simulink model "mcb_pmsm_foc_sensorless_dyno_f28379d"  (R2024b)
settings: Solver=FixedStepDiscrete  StartTime=0.0  StopTime=6  RelTol=1e-3  EnableMultiTasking=on
InitFcn:
  | mcb_pmsm_foc_sensorless_dyno_f28379d_datascript;
model workspace (MAT data in the model file):
  encoderResolution = 2000
  hallOffset = '0.5'
  indexOffset = 850
  polePairs = '4'
undefined symbols (not defined in the file or in its folder): acceleration, dataType, Down, GPTRIP1SEL, GPTRIP2SEL, inverter_motor1, inverter_motor2, PI_params_motor1, PI_params_motor2, pmsm_motor1, pmsm_motor2, PU_System_motor1, PU_System_motor2, PWM_frequency, SlidFCS_params, Speed_openLoop_PU, T_Ref_openLoop, target, Ts, Ts_motor, Ts_simulink, Ts_speed, TZ1, TZ2, Up, Vd_Ref_openLoop_PU
libraries: mcbcontrolslib x20, c2802xlib x14, simulink x8, c280xlib x7, slpidlib x5, c2837xDlib x5, mcbpositiondecoderlib x4, svdschedulerlib x3, mcbsensorlessestimatorlib x2, mcbpmsmnonlinearlib x2, autolibpmsmexterior x2, mcbplantlib x2
(part 1 of 4)
settings Model: ExtModeTrigDuration=8  Creator=The MathWorks, Inc.  LastModifiedBy=Eleonora
settings SolverCC: AlgebraicLoopSolver=TrustRegion
settings DataIOCC: LimitDataPoints=on  SaveFormat=Array  SaveOutput=off  SaveTime=off  ReturnWorkspaceOutputs=off
settings OptimizationCC: DefaultParameterBehavior=Inlined  DefaultUnderspecifiedDataType=single  OptimizeBlockIOStorage=off  BufferReuse=off  GlobalBufferReuse=off  ExpressionFolding=off  ExpressionDepthLimit=2147483647  LocalBlockOutputs=off  InitFltsAndDblsToZero=on  NoFixptDivByZeroProtection=on  EfficientFloat2IntCast=on  EfficientMapNaN2IntZero=off  LifeSpan=Inf  MaxStackSize=1024  OptimizeDataStoreBuffers=off  BusAssignmentInplaceUpdate=off  DenormalBehavior=FlushToZero  EfficientTunableParamExpr=on
settings DebuggingCC: ReadBeforeWriteMsg=DisableAll  WriteAfterWriteMsg=DisableAll  WriteAfterReadMsg=DisableAll  CheckSSInitialOutputMsg=off  SolverPrmCheckMsg=warning  InheritedTsInSrcMsg=none  MultiTaskDSMMsg=none  MultiTaskCondExecSysMsg=none  TasksWithSamePriorityMsg=none  SigSpecEnsureSampleTimeMsg=none  IntegerOverflowMsg=none  ParameterPrecisionLossMsg=none  FcnCallInpInsideContextMsg=warning  UnconnectedInputMsg=warning  UnconnectedOutputMsg=warning  UnconnectedLineMsg=warning  AllowSymbolicDim=off  StateNameClashWarn=warning  SFUnexpectedBacktrackingDiag=warning  SFNoUnconditionalDefaultTransitionDiag=warning  SFExecutionAtInitializationDiag=none  IntegerSaturationMsg=none  ArithmeticOperatorsInVariantConditions=warning
settings HardwareCC: ProdBitPerChar=16  ProdBitPerInt=16  ProdBitPerPointer=32  ProdBitPerSizeT=32  ProdBitPerPtrDiffT=32  ProdLargestAtomicInteger=Integer  ProdLargestAtomicFloat=None  ProdWordSize=16  ProdLongLongMode=on  ProdHWDeviceType=Texas Instruments->C2000  TargetBitPerChar=16  TargetBitPerInt=16  TargetBitPerPointer=16  TargetLargestAtomicInteger=Integer  TargetIntDivRoundTo=Zero  TargetEndianess=LittleEndian  TargetWordSize=16  TargetHWDeviceType=TI C2000
settings ModelReferenceCC: EnableRefExpFcnMdlSchedulingChecks=on  PropagateSignalLabelsOutOfModel=off
settings SFSimCC: SimUseLocalCustomCode=off  MATLABDynamicMemAlloc=off  CustomCodeUndefinedFunction=UseInterfaceOnly
settings RTWCC: Description=Embedded Coder  SystemTargetFile=ert.tlc  HardwareBoard=TI Delfino F28379D LaunchPad  TemplateMakefile=ert_default_tmf  GenerateReport=on  RTWUseLocalCustomCode=off  CustomHeaderCode="#include \"F2837xD_Ipc_drivers.h\""  Toolchain=Texas Instruments Code Composer Studio (C2000)  IncludeHyperlinkInReport=on  LaunchReport=on  GenerateTraceInfo=on  GenerateTraceReport=on  GenerateTraceReportSl=on  GenerateTraceReportSf=on  GenerateTraceReportEml=on  GPUComputeCapability=3.5  DLArmComputeVersion=19.05
settings CodeAppCC: IgnoreCustomStorageClasses=off  CustomSymbolStrType=$N$R$M  StateflowObjectComments=on  InternalIdentifier=Classic
settings ERTTargetCC: CodeReplacementLibrary=TI C28x  MultiwordLength=2048  ExtModeStaticAllocSize=10000  InlinedParameterPlacement=Hierarchical  ConvertIfToSwitch=off  SuppressUnreachableDefaultCases=off  MemSecPackage=tic2000demospkg  DynamicArrayContainerType=coder::array
settings ConfigComp: CovMetricSettings=dw  CovSaveCumulativeToWorkspaceVar=on  CovSaveSingleToWorkspaceVar=on  CovExternalEMLEnable=off  CovSFcnEnable=off

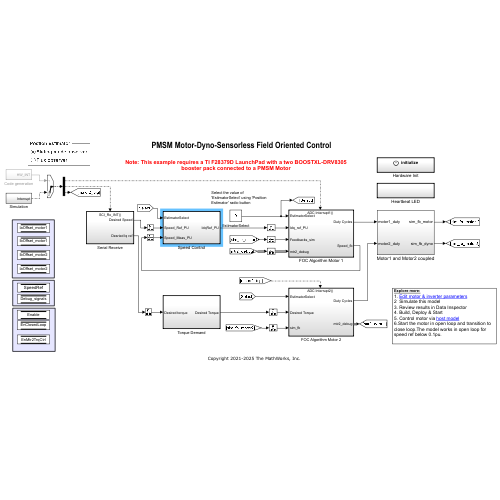
[thumbnail: Simulink's stored preview of the top-level diagram]
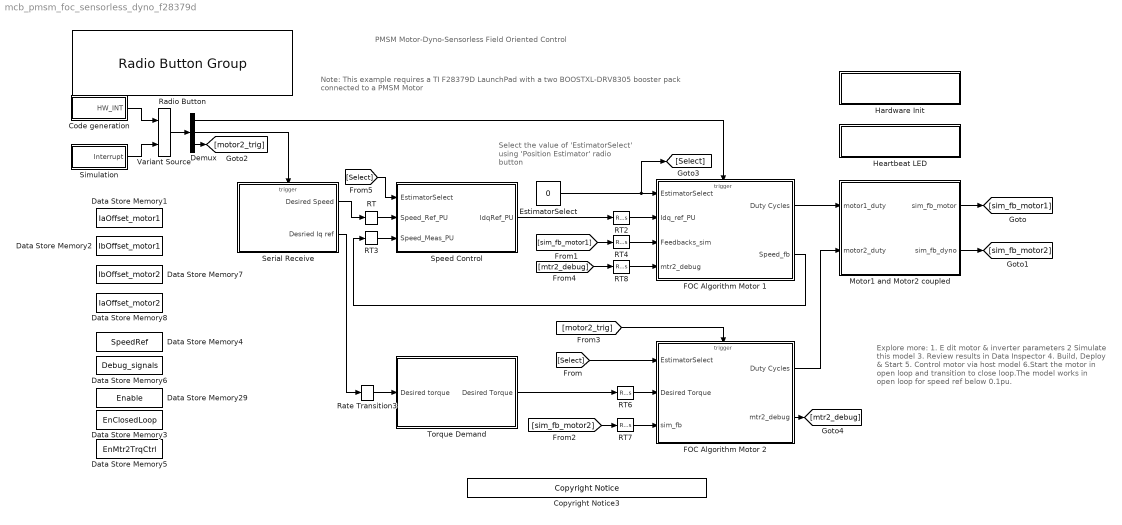
== system mcb_pmsm_foc_sensorless_dyno_f28379d ==
  note: PMSM Motor-Dyno-Sensorless Field Oriented Control
  note: Note: This example requires a TI F28379D LaunchPad with a two BOOSTXL-DRV8305
      | booster pack connected to a PMSM Motor
  note: Explore more:
      | 1. E dit motor & inverter parameters
      | 2 Simulate this model
      | 3. Review results in Data Inspector
      | 4. Build, Deploy & Start
      | 5. Control motor via host model
      | 6.Start the motor in open loop and transition to close loop.The model works in open loop for speed ref below 0.1pu.
  note: Select the value of 'EstimatorSelect' using 'Position Estimator' radio button
  Code generation : Subsystem
  Copyright Notice3 : demo_controls/Copyright Notice  year=2021  prod=tic2000
  Data Store Memory1 : DataStoreMemory  DataStoreName=IaOffset_motor1  ReadBeforeWriteMsg=warning  WriteAfterWriteMsg=warning  WriteAfterReadMsg=warning  InitialValue=inverter_motor1.CtSensAOffset  ShowAdditionalParam=off  OutDataTypeStr=uint16
  Data Store Memory2 : DataStoreMemory  DataStoreName=IbOffset_motor1  ReadBeforeWriteMsg=warning  WriteAfterWriteMsg=warning  WriteAfterReadMsg=warning  InitialValue=inverter_motor1.CtSensBOffset  ShowAdditionalParam=off  OutDataTypeStr=uint16
  Data Store Memory29 : DataStoreMemory  DataStoreName=Enable  ReadBeforeWriteMsg=warning  WriteAfterWriteMsg=warning  WriteAfterReadMsg=warning  ShowAdditionalParam=off  OutDataTypeStr=boolean
  Data Store Memory3 : DataStoreMemory  DataStoreName=EnClosedLoop  ReadBeforeWriteMsg=warning  WriteAfterWriteMsg=warning  WriteAfterReadMsg=warning  ShowAdditionalParam=off  OutDataTypeStr=boolean
  Data Store Memory4 : DataStoreMemory  DataStoreName=SpeedRef  InitialValue=0.1  ShowAdditionalParam=off
  Data Store Memory5 : DataStoreMemory  DataStoreName=EnMtr2TrqCtrl  ReadBeforeWriteMsg=warning  WriteAfterWriteMsg=warning  WriteAfterReadMsg=warning  ShowAdditionalParam=off  OutDataTypeStr=boolean
  Data Store Memory6 : DataStoreMemory  DataStoreName=Debug_signals  ReadBeforeWriteMsg=warning  WriteAfterWriteMsg=warning  WriteAfterReadMsg=warning  InitialValue=5  ShowAdditionalParam=off  OutDataTypeStr=uint16
  Data Store Memory7 : DataStoreMemory  DataStoreName=IbOffset_motor2  ReadBeforeWriteMsg=warning  WriteAfterWriteMsg=warning  WriteAfterReadMsg=warning  InitialValue=inverter_motor2.CtSensBOffset  ShowAdditionalParam=off  OutDataTypeStr=uint16
  Data Store Memory8 : DataStoreMemory  DataStoreName=IaOffset_motor2  ReadBeforeWriteMsg=warning  WriteAfterWriteMsg=warning  WriteAfterReadMsg=warning  InitialValue=inverter_motor2.CtSensBOffset  ShowAdditionalParam=off  OutDataTypeStr=uint16
  Demux : Demux  Outputs=3
  EstimatorSelect : Constant  Value=0
  FOC Algorithm Motor 1 : Subsystem
      settings: RTWSystemCode=Nonreusable function
  FOC Algorithm Motor 2 : Subsystem
      settings: RTWSystemCode=Nonreusable function
  Hardware Init : Subsystem  TreatAsAtomicUnit=on
  Heartbeat LED : Subsystem  TreatAsAtomicUnit=on
  Motor1 and Motor2 coupled : Subsystem
  RT : RateTransition  Deterministic=off  OutPortSampleTime=Ts_speed
  RT{2,4,6..8} (5 alike) : RateTransition  Deterministic=off
  RT3 : RateTransition  Deterministic=off  OutPortSampleTime=Ts_speed
  Radio Button : RadioButtonGroup  LabelPosition=Hide  SelectedLabel=Sliding mode observer  ButtonGroupName=Postion Estimator
      settings: Values={{'Sliding mode observer', 'Flux observer'}, [0 1]}
  Rate Transition3 : RateTransition  Deterministic=off  OutPortSampleTime=Ts_speed
  Serial Receive : Subsystem  SystemSampleTime=1e-3
  Simulation : Subsystem
  Speed Control : Subsystem  TreatAsAtomicUnit=on  SystemSampleTime=Ts_speed
  Torque Demand : Subsystem  TreatAsAtomicUnit=on  SystemSampleTime=Ts_speed
  Variant Source : VariantSource  VariantControlMode=sim codegen switching  OutputFunctionCall=on
  wires:
  Serial Receive/1(Desired Speed) -> RT/1
  RT3/1 -> Speed Control/3(Speed_Meas_PU)
  Speed Control/1(IdqRef_PU) -> RT2/1
  RT/1 -> Speed Control/2(Speed_Ref_PU)
  Motor1 and Motor2 coupled/1(sim_fb_motor) -> [sim_fb_motor1]
  FOC Algorithm Motor 1/1(Duty Cycles) -> Motor1 and Motor2 coupled/1(motor1_duty)
  [sim_fb_motor1] -> RT4/1
  RT2/1 -> FOC Algorithm Motor 1/2(Idq_ref_PU)
  EstimatorSelect/1 -> [Select], FOC Algorithm Motor 1/1(EstimatorSelect)
  Rate Transition3/1 -> Torque Demand/1(Desired torque)
  Serial Receive/2(Desried Iq ref) -> Rate Transition3/1
  FOC Algorithm Motor 2/1(Duty Cycles) -> Motor1 and Motor2 coupled/2(motor2_duty)
  Torque Demand/1(Desired Torque) -> RT6/1
  [motor2_trig] -> FOC Algorithm Motor 2/Trigger
  Demux/1 -> FOC Algorithm Motor 1/Trigger
  Simulation/1(Interrupt) -> Variant Source/2
  Code generation/1(HW_INT) -> Variant Source/1
  Demux/2 -> Serial Receive/Trigger
  Demux/3 -> [motor2_trig]
  Variant Source/1 -> Demux/1
  [sim_fb_motor2] -> RT7/1
  Motor1 and Motor2 coupled/2(sim_fb_dyno) -> [sim_fb_motor2]
  RT4/1 -> FOC Algorithm Motor 1/3(Feedbacks_sim)
  RT6/1 -> FOC Algorithm Motor 2/2(Desired Torque)
  RT7/1 -> FOC Algorithm Motor 2/3(sim_fb)
  FOC Algorithm Motor 1/2(Speed_fb) -> RT3/1
  FOC Algorithm Motor 2/2(mtr2_debug) -> [mtr2_debug]
  [mtr2_debug] -> RT8/1
  RT8/1 -> FOC Algorithm Motor 1/4(mtr2_debug)
  [Select] -> FOC Algorithm Motor 2/1(EstimatorSelect)
  [Select] -> Speed Control/1(EstimatorSelect)

== system mcb_pmsm_foc_sensorless_dyno_f28379d/Code generation ==
  HWI_ADCB1_INT : svdschedulerlib/Hardware Interrupt v2  ISRGroup=ADC - Analog to Digital Converter  ISRName=ADCA1_INT  ISRNumber=32  NumEventsToServe=1  EventsList={'on','EOC event','1';'off','Overflow event','2';'off','Custom event','3'}  SelectedEvents={'event1'}  TaskPriority=30  DisablePreemption=off  ClearInterruptFlagsAtEndOfEvent=on  InterruptDefinitionFile=$(TARGET_ROOT)/registry/interrupts/F2837xS_interrupts.xml  HardwareBoard=F2837x  EnableSimPort=off
      settings: LibrarySourceBlock=c2000lib/Scheduling/Hardware Interrupt
  HWI_ADCC1_INT : svdschedulerlib/Hardware Interrupt v2  ISRGroup=ADC - Analog to Digital Converter  ISRName=ADCA1_INT  ISRNumber=32  NumEventsToServe=1  EventsList={'on','EOC event','1';'off','Overflow event','2';'off','Custom event','3'}  SelectedEvents={'event1'}  TaskPriority=35  DisablePreemption=off  ClearInterruptFlagsAtEndOfEvent=on  InterruptDefinitionFile=$(TARGET_ROOT)/registry/interrupts/F2837xS_interrupts.xml  HardwareBoard=F2837x  EnableSimPort=off
      settings: LibrarySourceBlock=c2000lib/Scheduling/Hardware Interrupt
  HWI_SCIA_RX_INT : svdschedulerlib/Hardware Interrupt v2  ISRGroup=ADC - Analog to Digital Converter  ISRName=ADCA1_INT  ISRNumber=32  NumEventsToServe=1  EventsList={'on','EOC event','1';'off','Overflow event','2';'off','Custom event','3'}  SelectedEvents={'event1'}  TaskPriority=50  DisablePreemption=on  ClearInterruptFlagsAtEndOfEvent=on  InterruptDefinitionFile=$(TARGET_ROOT)/registry/interrupts/F2837xS_interrupts.xml  HardwareBoard=F2837x  EnableSimPort=off
      settings: LibrarySourceBlock=c2000lib/Scheduling/Hardware Interrupt
  Mux : Mux  Inputs=3
  HW_INT : Outport
  wires:
  HWI_ADCB1_INT/1 -> Mux/1
  HWI_SCIA_RX_INT/1 -> Mux/2
  HWI_ADCC1_INT/1 -> Mux/3
  Mux/1 -> HW_INT/1

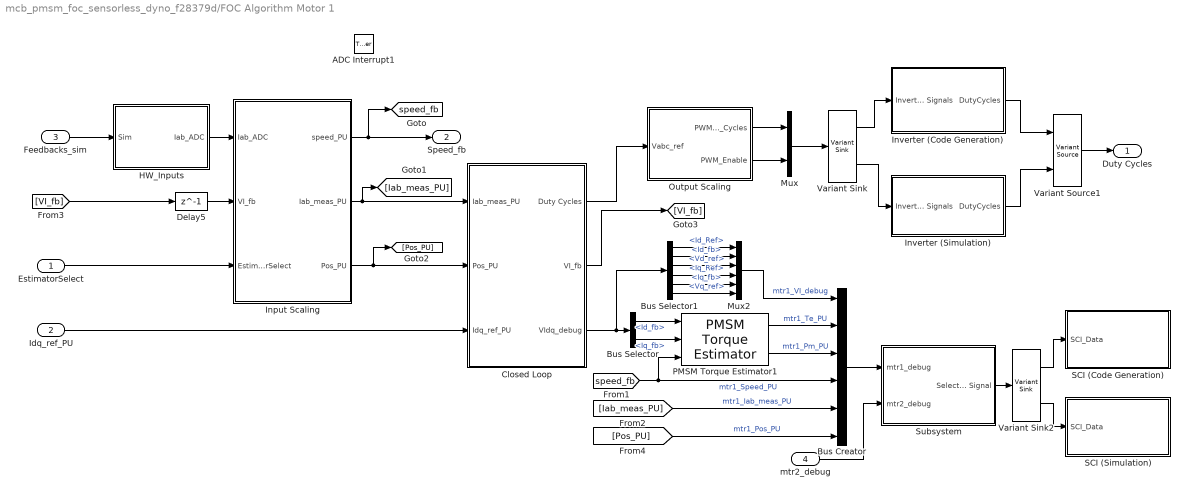
== system mcb_pmsm_foc_sensorless_dyno_f28379d/FOC Algorithm Motor 1 ==
  EstimatorSelect : Inport
  Idq_ref_PU : Inport  Port=2
  Feedbacks_sim : Inport  Port=3
  mtr2_debug : Inport  Port=4
  ADC Interrupt1 : TriggerPort  TriggerType=function-call  VariantControl=Variant  PortDimensions=1
  Bus Creator : BusCreator  Inputs=6
  Bus Selector : BusSelector  OutputSignals=Id_fb,Iq_fb
  Bus Selector1 : BusSelector  OutputSignals=Id_Ref,Id_fb,Vd_ref,Iq_Ref,Iq_fb,Vq_ref
  Closed Loop : Subsystem
  Delay5 : Delay  DelayLength=1
  HW_Inputs : Subsystem  Variant=on  VariantControlMode=sim codegen switching
  Input Scaling : Subsystem
  Inverter (Code Generation) : Subsystem
  Inverter (Simulation) : Subsystem
  Mux : Mux  Inputs=2
  Mux2 : Mux  Inputs=6
  Output Scaling : Subsystem
  PMSM Torque Estimator1 : mcbpmsmnonlinearlib/PMSM Torque Estimator  polePairs=pmsm_motor1.p  nonLinearityChoice=Linear model with lumped parameters  Ld=pmsm_motor1.Ld  Lq=pmsm_motor1.Lq  FluxPM=pmsm_motor1.FluxPM  idVec=[-40, -20, 0, 20]  iqVec=[-40, -20, 0, 20, 40]  LdTable=0.2e-3 * ones(4, 5)  LqTable=0.2e-3 * ones(4, 5)  FluxPMTable=6.4e-3 * ones(4, 5)  FluxDTable=[-1.6,-1.6,-1.6,-1.6,-1.6;2.4,2.4,2.4,2.4,2.4;6.4,6.4,6.4,6.4,6.4;10.4,10.4,10.4,10.4,10.4]*1e-3  FluxQTable=[-8,-4,0,4,8;-8,-4,0,4,8;-8,-4,0,4,8;-8,-4,0,4,8]*1e-3  Units=Per-Unit (PU)  V_base=PU_System_motor1.V_base  I_base=PU_System_motor1.I_base  N_base=PU_System_motor1.N_base  T_base=0.82227  P_base=445.3845  scaledTables=on
  SCI (Code Generation) : Subsystem
  SCI (Simulation) : Subsystem
  Subsystem : Subsystem
  Variant Sink : VariantSink  VariantControlMode=sim codegen switching
  Variant Sink2 : VariantSink  VariantControlMode=sim codegen switching
  Variant Source1 : VariantSource  VariantControlMode=sim codegen switching
  Duty Cycles : Outport  InitialOutput=0  VectorParamsAs1DForOutWhenUnconnected=off
  Speed_fb : Outport  Port=2  InitialOutput=0  VectorParamsAs1DForOutWhenUnconnected=off
  tag scope: speed_fb=global
  wires:
  HW_Inputs/1(Iab_ADC) -> Input Scaling/1(Iab_ADC)
  Delay5/1 -> Input Scaling/2(VI_fb)
  Subsystem/1(Selected Signal) -> Variant Sink2/1
  [VI_fb] -> Delay5/1
  Closed Loop/2(VI_fb) -> [VI_fb]
  Feedbacks_sim/1 -> HW_Inputs/1(Sim)
  Variant Source1/1 -> Duty Cycles/1
  Output Scaling/2(PWM_Enable) -> Mux/2
  Variant Sink/1 -> Inverter (Code Generation)/1(Inverter Signals)
  Variant Sink/2 -> Inverter (Simulation)/1(Inverter Signals)
  Mux/1 -> Variant Sink/1
  Variant Sink2/2 -> SCI (Simulation)/1(SCI_Data)
  Inverter (Code Generation)/1(DutyCycles) -> Variant Source1/1
  Inverter (Simulation)/1(DutyCycles) -> Variant Source1/2
  Variant Sink2/1 -> SCI (Code Generation)/1(SCI_Data)
  Output Scaling/1(PWM_Duty_Cycles) -> Mux/1
  Closed Loop/1(Duty Cycles) -> Output Scaling/1(Vabc_ref)
  Input Scaling/2(Iab_meas_PU) -> Closed Loop/1(Iab_meas_PU), [Iab_meas_PU]
  Idq_ref_PU/1 -> Closed Loop/3(Idq_ref_PU)
  Input Scaling/1(speed_PU) -> Speed_fb/1, [speed_fb]
  [Pos_PU] -> Bus Creator/6  "mtr1_Pos_PU"
  Bus Creator/1 -> Subsystem/1(mtr1_debug)
  PMSM Torque Estimator1/2 -> Bus Creator/3  "mtr1_Pm_PU"
  PMSM Torque Estimator1/1 -> Bus Creator/2  "mtr1_Te_PU"
  [speed_fb] -> PMSM Torque Estimator1/3, Bus Creator/4  "mtr1_Speed_PU"
  [Iab_meas_PU] -> Bus Creator/5  "mtr1_Iab_meas_PU"
  Bus Selector/1 -> PMSM Torque Estimator1/1  "<Id_fb>"
  Bus Selector/2 -> PMSM Torque Estimator1/2  "<Iq_fb>"
  Input Scaling/3(Pos_PU) -> Closed Loop/2(Pos_PU), [Pos_PU]
  mtr2_debug/1 -> Subsystem/2(mtr2_debug)
  Bus Selector1/5 -> Mux2/5  "<Iq_fb>"
  Bus Selector1/1 -> Mux2/1  "<Id_Ref>"
  Bus Selector1/2 -> Mux2/2  "<Id_fb>"
  Bus Selector1/3 -> Mux2/3  "<Vd_ref>"
  Bus Selector1/6 -> Mux2/6  "<Vq_ref>"
  Mux2/1 -> Bus Creator/1  "mtr1_VI_debug"
  Bus Selector1/4 -> Mux2/4  "<Iq_Ref>"
  Closed Loop/3(VIdq_debug) -> Bus Selector1/1, Bus Selector/1
  EstimatorSelect/1 -> Input Scaling/3(EstimatorSelect)

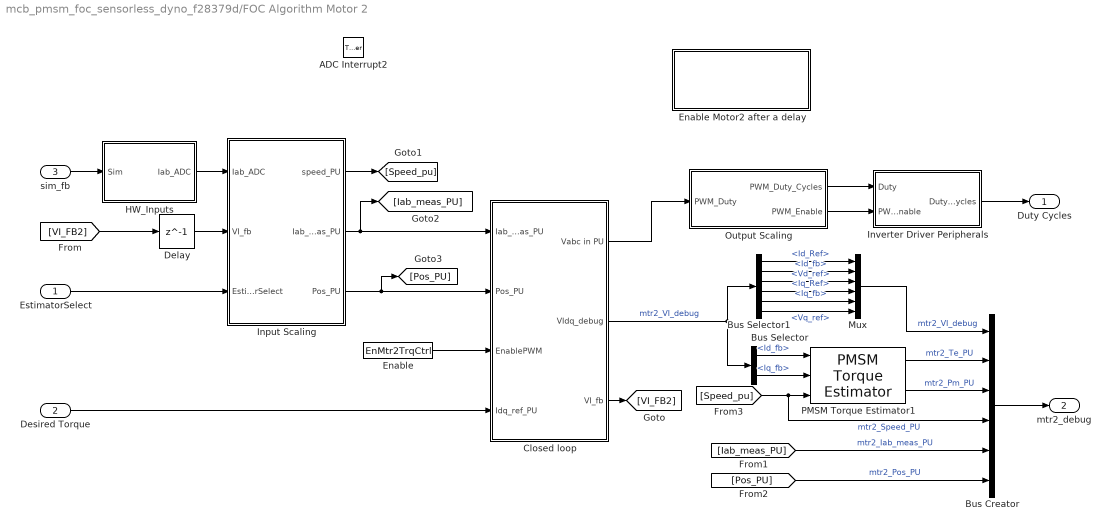
== system mcb_pmsm_foc_sensorless_dyno_f28379d/FOC Algorithm Motor 2 ==
  EstimatorSelect : Inport
  Desired Torque : Inport  Port=2
  sim_fb : Inport  Port=3
  ADC Interrupt2 : TriggerPort  TriggerType=function-call  VariantControl=Variant
  Bus Creator : BusCreator  Inputs=6
  Bus Selector : BusSelector  OutputSignals=Id_fb,Iq_fb
  Bus Selector1 : BusSelector  OutputSignals=Id_Ref,Id_fb,Vd_ref,Iq_Ref,Iq_fb,Vq_ref
  Closed loop : Subsystem
  Delay : Delay  DelayLength=1
  Enable : DataStoreRead  DataStoreName=EnMtr2TrqCtrl  IndexOptions=Index vector (dialog)  Indices=1  OutputSizes=1
  Enable Motor2 after a delay : Subsystem  Priority=10  Variant=on  VariantControlMode=sim codegen switching
  HW_Inputs : Subsystem  Variant=on  VariantControlMode=sim codegen switching
  Input Scaling : Subsystem
  Inverter Driver Peripherals : Subsystem
  Mux : Mux  Inputs=6
  Output Scaling : Subsystem
  PMSM Torque Estimator1 : mcbpmsmnonlinearlib/PMSM Torque Estimator  polePairs=pmsm_motor2.p  nonLinearityChoice=Linear model with lumped parameters  Ld=pmsm_motor2.Ld  Lq=pmsm_motor2.Lq  FluxPM=pmsm_motor2.FluxPM  idVec=[-40, -20, 0, 20]  iqVec=[-40, -20, 0, 20, 40]  LdTable=0.2e-3 * ones(4, 5)  LqTable=0.2e-3 * ones(4, 5)  FluxPMTable=6.4e-3 * ones(4, 5)  FluxDTable=[-1.6,-1.6,-1.6,-1.6,-1.6;2.4,2.4,2.4,2.4,2.4;6.4,6.4,6.4,6.4,6.4;10.4,10.4,10.4,10.4,10.4]*1e-3  FluxQTable=[-8,-4,0,4,8;-8,-4,0,4,8;-8,-4,0,4,8;-8,-4,0,4,8]*1e-3  Units=Per-Unit (PU)  V_base=PU_System_motor2.V_base  I_base=PU_System_motor2.I_base  N_base=PU_System_motor2.N_base  T_base=0.82227  P_base=445.3845  scaledTables=on
  Duty Cycles : Outport
  mtr2_debug : Outport  Port=2  VectorParamsAs1DForOutWhenUnconnected=off
  wires:
  Desired Torque/1 -> Closed loop/4(Idq_ref_PU)
  Closed loop/1(Vabc in PU) -> Output Scaling/1(PWM_Duty)
  Output Scaling/1(PWM_Duty_Cycles) -> Inverter Driver Peripherals/1(Duty)
  Output Scaling/2(PWM_Enable) -> Inverter Driver Peripherals/2(PWM_Enable)
  Inverter Driver Peripherals/1(Duty Cycles) -> Duty Cycles/1
  Closed loop/3(VI_fb) -> [VI_FB2]
  Input Scaling/3(Pos_PU) -> [Pos_PU], Closed loop/2(Pos_PU)
  [VI_FB2] -> Delay/1
  sim_fb/1 -> HW_Inputs/1(Sim)
  HW_Inputs/1(Iab_ADC) -> Input Scaling/1(Iab_ADC)
  Delay/1 -> Input Scaling/2(VI_fb)
  Input Scaling/2(Iab_meas_PU) -> [Iab_meas_PU], Closed loop/1(Iab_meas_PU)
  Input Scaling/1(speed_PU) -> [Speed_pu]
  EstimatorSelect/1 -> Input Scaling/3(EstimatorSelect)
  Bus Creator/1 -> mtr2_debug/1
  [Speed_pu] -> Bus Creator/4, PMSM Torque Estimator1/3  "mtr2_Speed_PU"
  Bus Selector/2 -> PMSM Torque Estimator1/2  "<Iq_fb>"
  Closed loop/2(VIdq_debug) -> Bus Selector1/1, Bus Selector/1  "mtr2_VI_debug"
  PMSM Torque Estimator1/1 -> Bus Creator/2  "mtr2_Te_PU"
  PMSM Torque Estimator1/2 -> Bus Creator/3  "mtr2_Pm_PU"
  Bus Selector/1 -> PMSM Torque Estimator1/1  "<Id_fb>"
  [Iab_meas_PU] -> Bus Creator/5  "mtr2_Iab_meas_PU"
  [Pos_PU] -> Bus Creator/6  "mtr2_Pos_PU"
  Bus Selector1/2 -> Mux/2  "<Id_fb>"
  Bus Selector1/1 -> Mux/1  "<Id_Ref>"
  Bus Selector1/3 -> Mux/3  "<Vd_ref>"
  Bus Selector1/4 -> Mux/4  "<Iq_Ref>"
  Bus Selector1/5 -> Mux/5  "<Iq_fb>"
  Bus Selector1/6 -> Mux/6  "<Vq_ref>"
  Mux/1 -> Bus Creator/1  "mtr2_VI_debug"
  Enable/1 -> Closed loop/3(EnablePWM)

== system mcb_pmsm_foc_sensorless_dyno_f28379d/Hardware Init ==
  Event Listener : EventListener  DisableCoverage=on  EventName=reset
  HW_Init : Subsystem  Variant=on  VariantControlMode=sim codegen switching

== system mcb_pmsm_foc_sensorless_dyno_f28379d/Heartbeat LED ==
  note: Heartbeat LED 1HZ
  Code generation : Subsystem
  RED_LED : Constant  OutDataTypeStr=uint16  SampleTime=0.5
  Simulation : Subsystem
  Variant Sink : VariantSink  VariantControlMode=sim codegen switching
  wires:
  RED_LED/1 -> Variant Sink/1
  Variant Sink/1 -> Code generation/1(In1)
  Variant Sink/2 -> Simulation/1(In1)

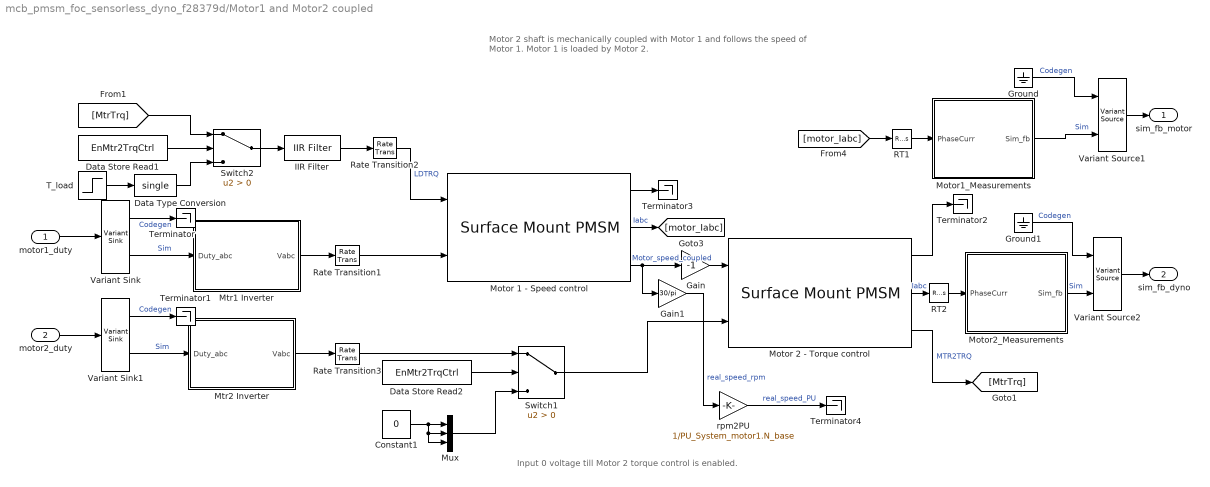
== system mcb_pmsm_foc_sensorless_dyno_f28379d/Motor1 and Motor2 coupled ==
  note: Motor 2 shaft is mechanically coupled with Motor 1
      | and follows the speed of Motor 1.
      |
      | Motor 1 is loaded by Motor 2.
  note: Input 0 voltage till Motor 2 torque control is enabled.
  motor1_duty : Inport
  motor2_duty : Inport  Port=2
  Constant1 : Constant  Value=0
  Data Store Read1 : DataStoreRead  DataStoreName=EnMtr2TrqCtrl  IndexOptions=Index vector (dialog)  Indices=1  OutputSizes=1
  Data Store Read2 : DataStoreRead  DataStoreName=EnMtr2TrqCtrl  IndexOptions=Index vector (dialog)  Indices=1  OutputSizes=1
  Data Type Conversion : DataTypeConversion  OutDataTypeStr=single  SaturateOnIntegerOverflow=off  RndMeth=Floor
  Gain : Gain  Gain=-1
  Gain1 : Gain  Gain=30/pi
  Ground : Ground
  Ground1 : Ground
  IIR Filter : mcbcontrolslib/IIR Filter  VariantControl=Low Pass Filter  VariantSelect=Low-pass  FilterConstantInputType=Specify via dialog  Filter_constant=0.0001  advancedSettings=off  Ts=50e-6  cutOff_freq=0.31834
  Motor 1 - Speed control : autolibpmsmexterior/Surface Mount PMSM  port_config=Torque  sim_type=Discrete  Ts=Ts_motor  P=pmsm_motor1.p  Rs=pmsm_motor1.Rs  Ldq_=pmsm_motor1.Ld  KConstText=Permanent flux linkage constant (lambda_pm):  lambda_pm=pmsm_motor1.FluxPM  Ke=159.9771  Kt=1.323  mechanical=[pmsm_motor1.J, pmsm_motor1.B, 0]  idq0=[0 0]  theta_init=0  omega_init=0  KConst=pmsm_motor1.FluxPM  lambda_pm_calc=pmsm_motor1.FluxPM  RefBlkName='autolibpmsmexterior/Surface Mount PMSM'  aMode=5  Ldq="[0.0002      0.0002]"
  Motor 2 - Torque control : autolibpmsmexterior/Surface Mount PMSM  port_config=Speed  sim_type=Discrete  Ts=Ts_motor  P=pmsm_motor2.p  Rs=pmsm_motor2.Rs  Ldq_=pmsm_motor2.Ld  KConstText=Permanent flux linkage constant (lambda_pm):  lambda_pm=pmsm_motor2.FluxPM  Ke=159.9771  Kt=1.323  mechanical=[0.0027, 4.924e-4, 0]  idq0=[0 0]  theta_init=0  omega_init=0  KConst=pmsm_motor2.FluxPM  lambda_pm_calc=pmsm_motor2.FluxPM  RefBlkName='autolibpmsmexterior/Surface Mount PMSM'  aMode=5  Ldq="[0.0002      0.0002]"
  Motor1_Measurements : Subsystem
  Motor2_Measurements : Subsystem
  Mtr1 Inverter : Subsystem
  Mtr2 Inverter : Subsystem
  Mux : Mux  Inputs=3
  RT1 : RateTransition  Deterministic=off  OutPortSampleTime=Ts_simulink
  RT2 : RateTransition  Deterministic=off  OutPortSampleTime=Ts_simulink
  Rate Transition1 : RateTransition  Deterministic=off  OutPortSampleTime=Ts_motor
  Rate Transition2 : RateTransition  Deterministic=off  OutPortSampleTime=Ts_motor
  Rate Transition3 : RateTransition  Deterministic=off  OutPortSampleTime=Ts_motor
  Switch1 : Switch  Criteria=u2 > Threshold  SaturateOnIntegerOverflow=off  InputSameDT=off
  Switch2 : Switch  Criteria=u2 > Threshold  SaturateOnIntegerOverflow=off  InputSameDT=off
  T_load : Step  Time=3  Before=0.05*pmsm_motor1.T_rated  After=0.4*pmsm_motor1.T_rated  SampleTime=Ts_simulink
  Terminator{,1..4} (5 alike) : Terminator
  Variant Sink : VariantSink  VariantControlMode=sim codegen switching
  Variant Sink1 : VariantSink  VariantControlMode=sim codegen switching
  Variant Source1 : VariantSource  VariantControlMode=sim codegen switching
  Variant Source2 : VariantSource  VariantControlMode=sim codegen switching
  rpm2PU : Gain  Gain=1/PU_System_motor1.N_base
  sim_fb_motor : Outport  VectorParamsAs1DForOutWhenUnconnected=off
  sim_fb_dyno : Outport  Port=2  VectorParamsAs1DForOutWhenUnconnected=off
  wires:
  motor1_duty/1 -> Variant Sink/1
  Variant Source1/1 -> sim_fb_motor/1
  Motor1_Measurements/1(Sim_fb) -> Variant Source1/2  "Sim"
  Ground/1 -> Variant Source1/1  "Codegen"
  Variant Sink/1 -> Terminator/1  "Codegen"
  Rate Transition1/1 -> Motor 1 - Speed control/2
  Mtr1 Inverter/1(Vabc) -> Rate Transition1/1
  Motor 1 - Speed control/3 -> Gain1/1, Gain/1  "Motor_speed_coupled"
  [motor_Iabc] -> RT1/1
  Motor 1 - Speed control/1 -> Terminator3/1
  Motor 1 - Speed control/2 -> [motor_Iabc]  "Iabc"
  Motor 2 - Torque control/2 -> RT2/1  "Iabc"
  Motor2_Measurements/1(Sim_fb) -> Variant Source2/2  "Sim"
  Mtr2 Inverter/1(Vabc) -> Rate Transition3/1
  Motor 2 - Torque control/3 -> [MtrTrq]  "MTR2TRQ"
  Variant Sink/2 -> Mtr1 Inverter/1(Duty_abc)  "Sim"
  Variant Sink1/2 -> Mtr2 Inverter/1(Duty_abc)  "Sim"
  Ground1/1 -> Variant Source2/1  "Codegen"
  Variant Source2/1 -> sim_fb_dyno/1
  motor2_duty/1 -> Variant Sink1/1
  Variant Sink1/1 -> Terminator1/1  "Codegen"
  Gain/1 -> Motor 2 - Torque control/1
  Rate Transition3/1 -> Switch1/1
  T_load/1 -> Data Type Conversion/1
  Data Store Read1/1 -> Switch2/2
  [MtrTrq] -> Switch2/1
  Switch1/1 -> Motor 2 - Torque control/2
  Mux/1 -> Switch1/3
  Data Store Read2/1 -> Switch1/2
  Constant1/1 -> Mux/2, Mux/3, Mux/1
  Motor 2 - Torque control/1 -> Terminator2/1
  Switch2/1 -> IIR Filter/1
  Data Type Conversion/1 -> Switch2/3
  RT1/1 -> Motor1_Measurements/1(PhaseCurr)
  RT2/1 -> Motor2_Measurements/1(PhaseCurr)
  IIR Filter/1 -> Rate Transition2/1
  Rate Transition2/1 -> Motor 1 - Speed control/1  "LDTRQ"
  Gain1/1 -> rpm2PU/1  "real_speed_rpm"
  rpm2PU/1 -> Terminator4/1  "real_speed_PU"

== system mcb_pmsm_foc_sensorless_dyno_f28379d/Serial Receive ==
  note: Simulation Input
  SCI_Rx_INT : TriggerPort  TriggerType=function-call  VariantControl=Variant
  Iq_Ref(A) : Step  Time=3  Before=1  After=0.7*pmsm_motor2.I_rated  OutDataTypeStr=single
  Parse SCI Rx : Subsystem
  Serial Receive : Subsystem  SystemSampleTime=1e-3
  Signal Editor : SignalEditorBlockLib/Signal Editor  Commented=on  FileName=speed-ref-signal.mat  ActiveScenario=Scenario  ActiveSignal=Signal 1  IsBus=off  OutputBusObjectStr=Bus: BusObject  SampleTime=-1  Interpolate=off  ZeroCross=off  OutputAfterFinalValue=Setting to zero  Unit=inherit  PreserveSignalName=on  ApplySigPropsToAllScenarios=on  ApplySigPropsToAllSignals=off
  Signal Packing : Subsystem
  Speed_Ref_CW (rpm) : Step  Time=T_Ref_openLoop  Before=Speed_openLoop_PU*pmsm_motor1.N_base  After=0.5*pmsm_motor1.N_base  OutDataTypeStr=single
  Variant Source1 : VariantSource  VariantControlMode=sim codegen switching
  Desired Speed : Outport
  Desried Iq ref : Outport  Port=2
  wires:
  Signal Packing/1(Data) -> Variant Source1/2  "Sim"
  Serial Receive/1(Rx) -> Variant Source1/1  "codegen"
  Variant Source1/1 -> Parse SCI Rx/1(Rx)
  Iq_Ref(A)/1 -> Signal Packing/2(IqRef)
  Parse SCI Rx/2(Desried Iq ref) -> Desried Iq ref/1
  Parse SCI Rx/1(Desired Speed) -> Desired Speed/1
  Speed_Ref_CW (rpm)/1 -> Signal Packing/1(Speedref)

== system mcb_pmsm_foc_sensorless_dyno_f28379d/Simulation ==
  Mux : Mux  Inputs=3
  Pulse Generator1 : DiscretePulseGenerator  PulseType=Time based  Period=Ts  PulseWidth=20  PhaseDelay=Ts
  Pulse Generator2 : DiscretePulseGenerator  PulseType=Time based  Period=Ts  PulseWidth=20
  SCI_Rx_INT : simulink/Ports & Subsystems/Function-Call Generator  sample_time=0.1  numberOfIterations=1  DisallowWideOutput=off
  Simulation1 : Subsystem
  Simulation2 : Subsystem
  Interrupt : Outport
  wires:
  Pulse Generator1/1 -> Simulation1/Trigger
  Mux/1 -> Interrupt/1
  SCI_Rx_INT/1 -> Mux/2
  Pulse Generator2/1 -> Simulation2/Trigger
  Simulation2/1(Interrupt) -> Mux/1
  Simulation1/1(Interrupt) -> Mux/3

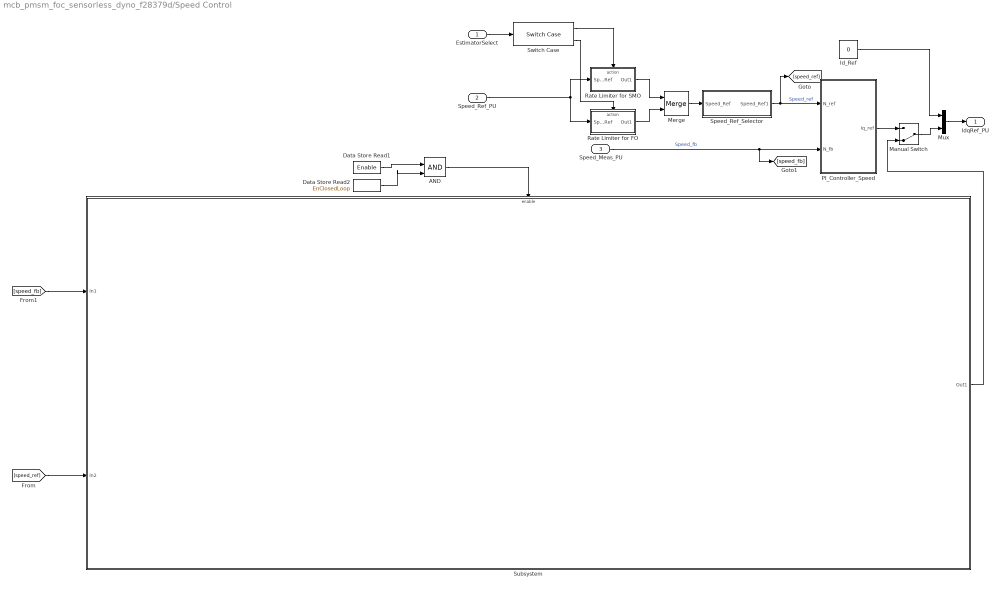
== system mcb_pmsm_foc_sensorless_dyno_f28379d/Speed Control ==
  EstimatorSelect : Inport
  Speed_Ref_PU : Inport  Port=2
  Speed_Meas_PU : Inport  Port=3
  AND : Logic  IconShape=distinctive  AllPortsSameDT=off  OutDataTypeStr=boolean
  Data Store Read2 : DataStoreRead  DataStoreName=EnClosedLoop  IndexOptions=Index vector (dialog)  Indices=1  OutputSizes=1
  Data Store Read1 : DataStoreRead  DataStoreName=Enable  IndexOptions=Index vector (dialog)  Indices=1  OutputSizes=1
  Id_Ref : Constant  Value=0  OutDataTypeStr=dataType
  Manual Switch : ManualSwitch  CurrentSetting=0
  Merge : Merge
  Mux : Mux  Inputs=2
  PI_Controller_Speed : Subsystem
  Rate Limiter for FO : Subsystem  TreatAsAtomicUnit=on
  Rate Limiter for SMO : Subsystem  TreatAsAtomicUnit=on
  Speed_Ref_Selector : Subsystem
  Subsystem : Subsystem
  Switch Case : SwitchCase  CaseConditions={0,1}  ShowDefaultCase=off
  IdqRef_PU : Outport  VectorParamsAs1DForOutWhenUnconnected=off
  wires:
  Speed_Meas_PU/1 -> [speed_fb], PI_Controller_Speed/2(N_fb)  "Speed_fb"
  Id_Ref/1 -> Mux/1
  Mux/1 -> IdqRef_PU/1
  Speed_Ref_PU/1 -> Rate Limiter for FO/1(Speed_Ref), Rate Limiter for SMO/1(Speed_Ref)
  Speed_Ref_Selector/1(Speed_Ref1) -> [speed_ref], PI_Controller_Speed/1(N_ref)  "Speed_ref"
  Merge/1 -> Speed_Ref_Selector/1(Speed_Ref)
  Switch Case/1 -> Rate Limiter for SMO/Action
  Switch Case/2 -> Rate Limiter for FO/Action
  EstimatorSelect/1 -> Switch Case/1
  Rate Limiter for FO/1(Out1) -> Merge/2
  Rate Limiter for SMO/1(Out1) -> Merge/1
  PI_Controller_Speed/1(Iq_ref) -> Manual Switch/1
  Manual Switch/1 -> Mux/2
  [speed_fb] -> Subsystem/1(In1)
  [speed_ref] -> Subsystem/2(In2)
  Subsystem/1(Out1) -> Manual Switch/2
  AND/1 -> Subsystem/Enable
  Data Store Read1/1 -> AND/1
  Data Store Read2/1 -> AND/2

== system mcb_pmsm_foc_sensorless_dyno_f28379d/Torque Demand ==
  Desired torque : Inport
  IIR Filter : mcbcontrolslib/IIR Filter  VariantControl=Low Pass Filter  VariantSelect=Low-pass  FilterConstantInputType=Specify via dialog  Filter_constant=0.01*(Ts_speed/Ts)  advancedSettings=off  Ts=50e-6  cutOff_freq=795.7747
  Id_ref_PU : Constant  Value=0  OutDataTypeStr=dataType
  Mux : Mux  Inputs=2
  Desired Torque : Outport
  wires:
  Id_ref_PU/1 -> Mux/1
  Mux/1 -> IIR Filter/1
  Desired torque/1 -> Mux/2
  IIR Filter/1 -> Desired Torque/1

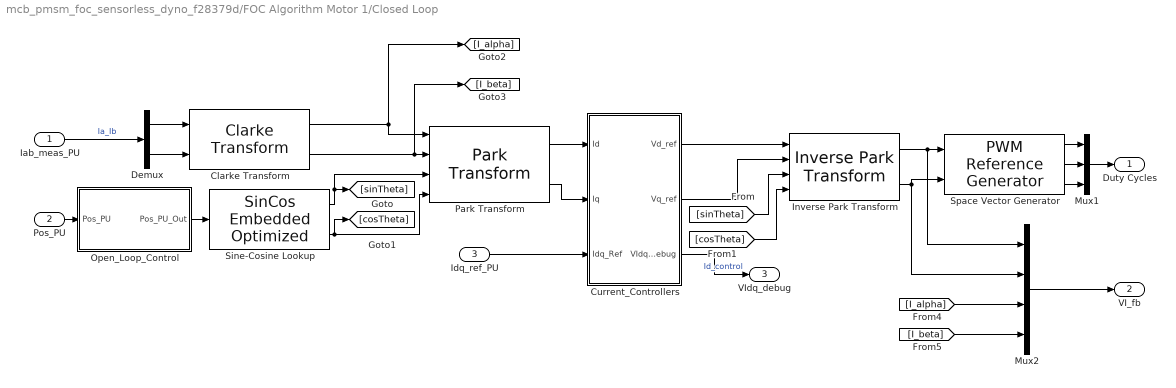
== system mcb_pmsm_foc_sensorless_dyno_f28379d/FOC Algorithm Motor 1/Closed Loop ==
  Iab_meas_PU : Inport
  Pos_PU : Inport  Port=2
  Idq_ref_PU : Inport  Port=3
  Clarke Transform : mcbcontrolslib/Clarke Transform  VariantControl=Variant2  PhaseInput=Two inputs  EnPowerInv=off
  Current_Controllers : Subsystem
  Demux : Demux  Outputs=2
  Inverse Park Transform : mcbcontrolslib/Inverse Park Transform  PhaseInput=Two inputs  AxisAlignment=D-axis  ThetaInput=Sine and Cosine electrical position  AngleInput=Per-unit  N_points=1024
  Mux1 : Mux  Inputs=3
  Mux2 : Mux
  Open_Loop_Control : Subsystem
  Park Transform : mcbcontrolslib/Park Transform  PhaseInput=Two inputs  AxisAlignment=D-axis  ThetaInput=Sine and Cosine electrical position  AngleInput=Per-unit  N_points=1024
  Sine-Cosine Lookup : mcbcontrolslib/SinCos Embedded Optimized  LabelModeActiveChoice=MCB_Sin  OptforProc=off  ApproximationMethod=None  UserApproxMethod=Lookup  ApproxStatus=None  InterpMethod=Linear point-slope  NumberOfDataPoints=16  NumberOfIterations=11  RemoveProtectionAgainstOutOfRangeInput=off  TableDataTypeStr=Inherit: Inherit via input  AngleInput=Per-unit  ThetaDataType=single  N_points=1024  DatatypeInput=Inherit from input  Datatype=single
  Space Vector Generator : mcbcontrolslib/PWM Reference Generator  inSignal=Valphabeta  modType=SVM: space vector modulation
  Duty Cycles : Outport  VectorParamsAs1DForOutWhenUnconnected=off
  VI_fb : Outport  Port=2  VectorParamsAs1DForOutWhenUnconnected=off
  VIdq_debug : Outport  Port=3  VectorParamsAs1DForOutWhenUnconnected=off
  wires:
  Current_Controllers/1(Vd_ref) -> Inverse Park Transform/1
  [cosTheta] -> Inverse Park Transform/4
  [I_beta] -> Mux2/4
  Inverse Park Transform/2 -> Space Vector Generator/2, Mux2/2
  Inverse Park Transform/1 -> Space Vector Generator/1, Mux2/1
  [sinTheta] -> Inverse Park Transform/3
  Mux2/1 -> VI_fb/1
  Clarke Transform/1 -> Park Transform/1, [I_alpha]
  Current_Controllers/2(Vq_ref) -> Inverse Park Transform/2
  Clarke Transform/2 -> [I_beta], Park Transform/2
  Sine-Cosine Lookup/1 -> Park Transform/3, [sinTheta]
  [I_alpha] -> Mux2/3
  Space Vector Generator/1 -> Mux1/1
  Space Vector Generator/3 -> Mux1/3
  Mux1/1 -> Duty Cycles/1
  Sine-Cosine Lookup/2 -> Park Transform/4, [cosTheta]
  Space Vector Generator/2 -> Mux1/2
  Demux/1 -> Clarke Transform/1
  Demux/2 -> Clarke Transform/2
  Iab_meas_PU/1 -> Demux/1  "Ia_Ib"
  Idq_ref_PU/1 -> Current_Controllers/3(Idq_Ref)
  Pos_PU/1 -> Open_Loop_Control/1(Pos_PU)
  Current_Controllers/3(VIdq_debug) -> VIdq_debug/1  "Id_control"
  Open_Loop_Control/1(Pos_PU_Out) -> Sine-Cosine Lookup/1
  Park Transform/1 -> Current_Controllers/1(Id)
  Park Transform/2 -> Current_Controllers/2(Iq)

== system mcb_pmsm_foc_sensorless_dyno_f28379d/FOC Algorithm Motor 1/HW_Inputs ==
  Sim : Inport
  Sensor Driver Blocks (codegen) : Subsystem  VariantControl=(codegen)
  Sensor Driver Blocks (sim) : Subsystem  VariantControl=(sim)
  Iab_ADC : Outport

== system mcb_pmsm_foc_sensorless_dyno_f28379d/FOC Algorithm Motor 1/Input Scaling ==
  note: Current Measurements
  Iab_ADC : Inport
  VI_fb : Inport  Port=2
  EstimatorSelect : Inport  Port=3
  Calculate Phase Currents : Subsystem
  Calculate position and speed : Subsystem
  Demux : Demux  Outputs=2
  speed_PU : Outport
  Iab_meas_PU : Outport  Port=2
  Pos_PU : Outport  Port=3
  wires:
  Calculate Phase Currents/1(Iab_meas_PU) -> Iab_meas_PU/1  "Iab_fb_PU"
  Iab_ADC/1 -> Demux/1
  Calculate position and speed/2(speed_PU) -> speed_PU/1
  Calculate position and speed/1(Pos_PU) -> Pos_PU/1
  VI_fb/1 -> Calculate position and speed/2(VI_fb)
  EstimatorSelect/1 -> Calculate position and speed/1(EstimatorSelect)
  Demux/1 -> Calculate Phase Currents/1(Ia_ADC)
  Demux/2 -> Calculate Phase Currents/2(Ib_ADC)

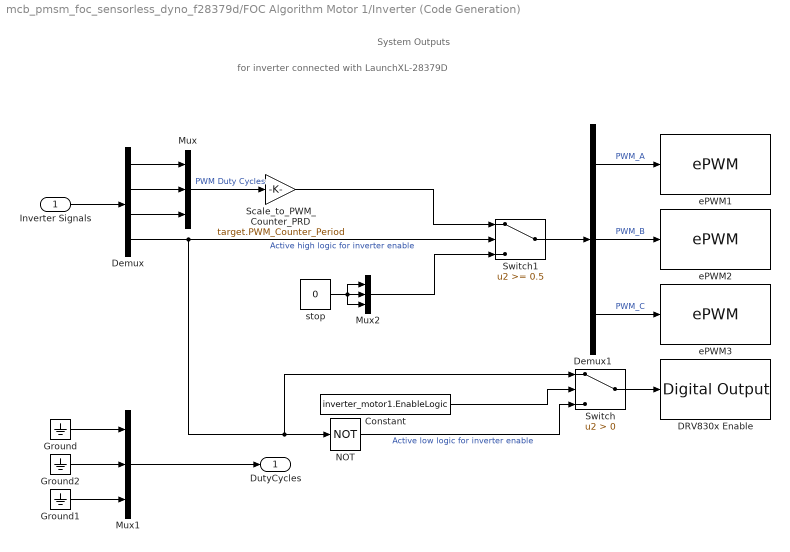
== system mcb_pmsm_foc_sensorless_dyno_f28379d/FOC Algorithm Motor 1/Inverter (Code Generation) ==
  note: for inverter connected with LaunchXL-28379D
  note: System Outputs
  Inverter Signals : Inport
  Constant : Constant  Value=inverter_motor1.EnableLogic
  DRV830x Enable : c2837xDlib/Digital Output  GPIO_Number=GPIO120~GPIO127  GPIO_Bit0=off  GPIO_BIT0_Toggle=off  GPIO_Bit1=off  GPIO_BIT1_Toggle=off  GPIO_Bit2=off  GPIO_BIT2_Toggle=off  GPIO_Bit3=off  GPIO_BIT3_Toggle=off  GPIO_Bit4=on  GPIO_BIT4_Toggle=off  GPIO_Bit5=off  GPIO_BIT5_Toggle=off  GPIO_Bit6=off  GPIO_BIT6_Toggle=off  GPIO_Bit7=off  GPIO_BIT7_Toggle=off
  Demux : Demux
  Demux1 : Demux  Outputs=3
  Ground : Ground
  Ground1 : Ground
  Ground2 : Ground
  Mux : Mux  Inputs=3
  Mux1 : Mux  Inputs=3
  Mux2 : Mux  Inputs=3
  NOT : Logic  Operator=NOT  IconShape=distinctive  AllPortsSameDT=off  OutDataTypeStr=boolean
  Scale_to_PWM_Counter_PRD : Gain  Gain=target.PWM_Counter_Period  OutDataTypeStr=uint16  RndMeth=Simplest
  Switch : Switch  Criteria=u2 > Threshold  SaturateOnIntegerOverflow=off  InputSameDT=off
  Switch1 : Switch  Threshold=0.5  SaturateOnIntegerOverflow=off  InputSameDT=off
  ePWM1 : c2802xlib/ePWM  PwmType=C2000_Type4  useModule=ePWM1  ePWMxLINKTBPRD=Not Linked  periodUnits=Clock cycles  timerSource=Specify via dialog  timerPeriod_clk=target.PWM_Counter_Period  timerPeriod_sec=0.0001  tbshadow=Counter equals to zero  countingMode=Up-Down  phaseActiveEnable=Disable  phaseDirection=Count down after sync  phaseActive=0  synchronizationEnable=off  dcaevt1Sync=off  dcbevt1Sync=off  synchronizationOption=Counter equals to zero (CTR=Zero)  dcbevt1SyncOut=off  dcaevt1SyncOut=off  cmpdSyncOut=off  cmpcSyncOut=off  cmpbSyncOut=off  zeroSyncOut=on  swfSyncOut=off  perSynchronizationOption=Counter equals to period (CTR=PRD)  clockPrescale=1  HSclockPrescale=1  enswap=off  ePWMxAStatus=on  ePWMxAactionLogic1=Do nothing  ePWMxAactionLogic2=Do nothing  ePWMxAactionLogic3=Clear  ePWMxAactionLogic4=Set  ePWMxAactionLogic5=Do nothing  ePWMxAactionLogic6=Do nothing  ePWMxACSFenable=off  ePWMxACSFvalue=Forcing disable  ePWMxASFreload=Zero  ePWMxBStatus=off  ePWMxBactionLogic1=Set  ePWMxBactionLogic2=Clear  ePWMxBactionLogic3=Do nothing  ePWMxBactionLogic4=Do nothing  ePWMxBactionLogic5=Clear  ePWMxBactionLogic6=Set  ePWMxBCSFenable=off  ePWMxBCSFvalue=Forcing disable  ePWMxBSFreload=Zero  ePWNxBOutWay=off  ePWMxLINKCMPA=Not Linked  CMPAUnits=Clock cycles  CMPASource=Input port  CMPAValue_per=50  CMPAValue_clk=floor(target.PWM_Counter_Period/2+1)  enCMPAshadow=Counter equals to zero (CTR=Zero)  ePWMxLINKCMPB=Not Linked  CMPBUnits=Clock cycles  CMPBSource=Specify via dialog  CMPBValue_per=50  CMPBValue_clk=floor(target.PWM_Counter_Period/2+1)  enCMPBshadow=Counter equals to zero (CTR=Zero)  ePWMxLINKCMPC=Not Linked  CMPCUnits=Clock cycles  CMPCSource=Specify via dialog  CMPCValue_per=50  CMPCValue_clk=32000  enCMPCshadow=Counter equals to zero (CTR=Zero)  ePWMxLINKCMPD=Not Linked  CMPDUnits=Clock cycles  CMPDSource=Specify via dialog  CMPDValue_per=50  CMPDValue_clk=32000  enCMPDshadow=Counter equals to zero (CTR=Zero)  enableDBePWMxA=on  enableDBePWMxB=on  enhalfcycle=off  DBpolarity=Active high complementary (AHC)  DBedgeDelay=Positive  DBSource_ePWMxA=ePWMxA  DBSource_ePWMxB=ePWMxA  DBPeriodUnits=Clock cycles  DBperiodSource=Specify via dialog  REDperiod=15  FEDperiod=15  REDperiod_sec=0  FEDperiod_sec=0  LoadModeDBRED=Immediate without using shadow  LoadModeDBFED=Immediate without using shadow  adcstartModuleA=on  adcrequestEventA=First event  adcstartEventA=Digital Compare Module A Event 1 start of conversion (DCAEVT1.soc)  adcstartEventA_type2=Counter equals to period (CTR=PRD)  adcstartModuleB=off  adcrequestEventB=First event  adcstartEventB=Counter equals to zero (CTR=Zero)  adcstartEventB_type2=Counter equals to zero (CTR=Zero)  intEn=off  intPrd=First event  intSel=Counter equals to zero (CTR=Zero)  intSel_type2=Counter equals to zero (CTR=Zero)  hrpe=off  enHRPWM=off  HRPWM_LoadMode=Counter equals to period (CTR=PRD)  HRPWM_CTLMode=Duty or Period control mode  HRPWM_EDGMode=Both edge  hrpeb=off  enHRPWMB=off  HRPWM_LoadModeB=Counter equals to zero (CTR=ZERO)  HRPWM_CTLModeB=Duty or Period control mode  HRPWM_EDGModeB=Both edge  enHRDBRED=off  enHRDBFED=off  enSFO=on  enautoconv=on  chopperEnable=off  chopperFrequency=1  chopperFirstwidth=1  chopperDuty=12.5%  tripZonesource=Specify via dialog  tzselOSHT1=off  tzselOSHT2=off  tzselOSHT3=off  tzselOSHT4=off  tzselOSHT5=off  tzselOSHT6=off  tzselOSHDCAEV1=off  tzselOSHDCBEV1=off  tzselCBC1=off  tzselCBC2=off  tzselCBC3=off  tzselCBC4=off  tzselCBC5=off  tzselCBC6=off  tzselCBCDCAEV2=off  tzselCBCDCBEV2=off  enTzOstIntr=off  enTzCbcIntr=off  enTzDCAEVT1Intr=off  enTzDCAEVT2Intr=off  enTzDCBEVT1Intr=off  enTzDCBEVT2Intr=off  tzclrCBCLatch=Counter equals to zero (CTR=Zero)  ePWMxAforced=No action  ePWMxBforced=No action  DCAEVT1forced=No action  DCBEVT1forced=No action  DCAEVT2forced=No action  DCBEVT2forced=No action  dcah=Trip Zone 1 input (TZ1)  dcal=Trip Zone 2 input (TZ2)  dcbh=Trip Zone 1 input (TZ1)  dcbl=Trip Zone 2 input (TZ2)  dcah_type2=GPTRIP1SEL/(TZ1)  dcal_type2=GPTRIP2SEL/(TZ2)  dcbh_type2=GPTRIP1SEL/(TZ1)  dcbl_type2=GPTRIP2SEL/(TZ2)  gendcaevt1=Event disabled  gendcaevt2=Event disabled  gendcbevt1=Event disabled  gendcbevt2=Event disabled  dcaevt1src=DCAEVT1 with sync  dcaevt2src=DCAEVT2 with sync  dcbevt1src=DCBEVT1 with sync  dcbevt2src=DCBEVT2 with sync  pulsesel=Counter equals to zero (CTR=Zero)  blankinv=off  blankoffset=0  blankwidth=0  evsrcsel=Filtered version of DCAEVT1 (DCAEVT1FILT)  encape=off
  ePWM2 : c2802xlib/ePWM  PwmType=C2000_Type4  useModule=ePWM2  ePWMxLINKTBPRD=Not Linked  periodUnits=Clock cycles  timerSource=Specify via dialog  timerPeriod_clk=target.PWM_Counter_Period  timerPeriod_sec=0.0001  tbshadow=Counter equals to zero  countingMode=Up-Down  phaseActiveEnable=Set counter to phase value specified via dialog  phaseDirection=Count up after sync  phaseActive=0  synchronizationEnable=off  dcaevt1Sync=off  dcbevt1Sync=off  synchronizationOption=Pass through (EPWMxSYNCI or SWFSYNC)  dcbevt1SyncOut=off  dcaevt1SyncOut=off  cmpdSyncOut=off  cmpcSyncOut=off  cmpbSyncOut=off  zeroSyncOut=off  swfSyncOut=on  perSynchronizationOption=Counter equals to period (CTR=PRD)  clockPrescale=1  HSclockPrescale=1  enswap=off  ePWMxAStatus=on  ePWMxAactionLogic1=Do nothing  ePWMxAactionLogic2=Do nothing  ePWMxAactionLogic3=Clear  ePWMxAactionLogic4=Set  ePWMxAactionLogic5=Do nothing  ePWMxAactionLogic6=Do nothing  ePWMxACSFenable=off  ePWMxACSFvalue=Forcing disable  ePWMxASFreload=Zero  ePWMxBStatus=off  ePWMxBactionLogic1=Set  ePWMxBactionLogic2=Clear  ePWMxBactionLogic3=Do nothing  ePWMxBactionLogic4=Do nothing  ePWMxBactionLogic5=Clear  ePWMxBactionLogic6=Set  ePWMxBCSFenable=off  ePWMxBCSFvalue=Forcing disable  ePWMxBSFreload=Zero  ePWNxBOutWay=off  ePWMxLINKCMPA=Not Linked  CMPAUnits=Clock cycles  CMPASource=Input port  CMPAValue_per=50  CMPAValue_clk=floor(target.PWM_Counter_Period/2+1)  enCMPAshadow=Counter equals to zero (CTR=Zero)  ePWMxLINKCMPB=Not Linked  CMPBUnits=Clock cycles  CMPBSource=Specify via dialog  CMPBValue_per=50  CMPBValue_clk=floor(target.PWM_Counter_Period/2+1)  enCMPBshadow=Counter equals to zero (CTR=Zero)  ePWMxLINKCMPC=Not Linked  CMPCUnits=Clock cycles  CMPCSource=Specify via dialog  CMPCValue_per=50  CMPCValue_clk=32000  enCMPCshadow=Counter equals to zero (CTR=Zero)  ePWMxLINKCMPD=Not Linked  CMPDUnits=Clock cycles  CMPDSource=Specify via dialog  CMPDValue_per=50  CMPDValue_clk=32000  enCMPDshadow=Counter equals to zero (CTR=Zero)  enableDBePWMxA=on  enableDBePWMxB=on  enhalfcycle=off  DBpolarity=Active high complementary (AHC)  DBedgeDelay=Positive  DBSource_ePWMxA=ePWMxA  DBSource_ePWMxB=ePWMxA  DBPeriodUnits=Clock cycles  DBperiodSource=Specify via dialog  REDperiod=15  FEDperiod=15  REDperiod_sec=0  FEDperiod_sec=0  LoadModeDBRED=Immediate without using shadow  LoadModeDBFED=Immediate without using shadow  adcstartModuleA=off  adcrequestEventA=First event  adcstartEventA=Digital Compare Module A Event 1 start of conversion (DCAEVT1.soc)  adcstartEventA_type2=Counter equals to period (CTR=PRD)  adcstartModuleB=off  adcrequestEventB=First event  adcstartEventB=Counter equals to zero (CTR=Zero)  adcstartEventB_type2=Counter equals to zero (CTR=Zero)  intEn=off  intPrd=First event  intSel=Counter equals to zero (CTR=Zero)  intSel_type2=Counter equals to zero (CTR=Zero)  hrpe=off  enHRPWM=off  HRPWM_LoadMode=Counter equals to period (CTR=PRD)  HRPWM_CTLMode=Duty or Period control mode  HRPWM_EDGMode=Both edge  hrpeb=off  enHRPWMB=off  HRPWM_LoadModeB=Counter equals to zero (CTR=ZERO)  HRPWM_CTLModeB=Duty or Period control mode  HRPWM_EDGModeB=Both edge  enHRDBRED=off  enHRDBFED=off  enSFO=on  enautoconv=on  chopperEnable=off  chopperFrequency=1  chopperFirstwidth=1  chopperDuty=12.5%  tripZonesource=Specify via dialog  tzselOSHT1=off  tzselOSHT2=off  tzselOSHT3=off  tzselOSHT4=off  tzselOSHT5=off  tzselOSHT6=off  tzselOSHDCAEV1=off  tzselOSHDCBEV1=off  tzselCBC1=off  tzselCBC2=off  tzselCBC3=off  tzselCBC4=off  tzselCBC5=off  tzselCBC6=off  tzselCBCDCAEV2=off  tzselCBCDCBEV2=off  enTzOstIntr=off  enTzCbcIntr=off  enTzDCAEVT1Intr=off  enTzDCAEVT2Intr=off  enTzDCBEVT1Intr=off  enTzDCBEVT2Intr=off  tzclrCBCLatch=Counter equals to zero (CTR=Zero)  ePWMxAforced=No action  ePWMxBforced=No action  DCAEVT1forced=No action  DCBEVT1forced=No action  DCAEVT2forced=No action  DCBEVT2forced=No action  dcah=Trip Zone 1 input (TZ1)  dcal=Trip Zone 2 input (TZ2)  dcbh=Trip Zone 1 input (TZ1)  dcbl=Trip Zone 2 input (TZ2)  dcah_type2=GPTRIP1SEL/(TZ1)  dcal_type2=GPTRIP2SEL/(TZ2)  dcbh_type2=GPTRIP1SEL/(TZ1)  dcbl_type2=GPTRIP2SEL/(TZ2)  gendcaevt1=Event disabled  gendcaevt2=Event disabled  gendcbevt1=Event disabled  gendcbevt2=Event disabled  dcaevt1src=DCAEVT1 with sync  dcaevt2src=DCAEVT2 with sync  dcbevt1src=DCBEVT1 with sync  dcbevt2src=DCBEVT2 with sync  pulsesel=Counter equals to zero (CTR=Zero)  blankinv=off  blankoffset=0  blankwidth=0  evsrcsel=Filtered version of DCAEVT1 (DCAEVT1FILT)  encape=off
  ePWM3 : c2802xlib/ePWM  PwmType=C2000_Type4  useModule=ePWM3  ePWMxLINKTBPRD=Not Linked  periodUnits=Clock cycles  timerSource=Specify via dialog  timerPeriod_clk=target.PWM_Counter_Period  timerPeriod_sec=0.0001  tbshadow=Counter equals to zero  countingMode=Up-Down  phaseActiveEnable=Set counter to phase value specified via dialog  phaseDirection=Count up after sync  phaseActive=0  synchronizationEnable=off  dcaevt1Sync=off  dcbevt1Sync=off  synchronizationOption=Pass through (EPWMxSYNCI or SWFSYNC)  dcbevt1SyncOut=off  dcaevt1SyncOut=off  cmpdSyncOut=off  cmpcSyncOut=off  cmpbSyncOut=off  zeroSyncOut=off  swfSyncOut=on  perSynchronizationOption=Counter equals to period (CTR=PRD)  clockPrescale=1  HSclockPrescale=1  enswap=off  ePWMxAStatus=on  ePWMxAactionLogic1=Do nothing  ePWMxAactionLogic2=Do nothing  ePWMxAactionLogic3=Clear  ePWMxAactionLogic4=Set  ePWMxAactionLogic5=Do nothing  ePWMxAactionLogic6=Do nothing  ePWMxACSFenable=off  ePWMxACSFvalue=Forcing disable  ePWMxASFreload=Zero  ePWMxBStatus=off  ePWMxBactionLogic1=Set  ePWMxBactionLogic2=Clear  ePWMxBactionLogic3=Do nothing  ePWMxBactionLogic4=Do nothing  ePWMxBactionLogic5=Clear  ePWMxBactionLogic6=Set  ePWMxBCSFenable=off  ePWMxBCSFvalue=Forcing disable  ePWMxBSFreload=Zero  ePWNxBOutWay=off  ePWMxLINKCMPA=Not Linked  CMPAUnits=Clock cycles  CMPASource=Input port  CMPAValue_per=50  CMPAValue_clk=floor(target.PWM_Counter_Period/2+1)  enCMPAshadow=Counter equals to zero (CTR=Zero)  ePWMxLINKCMPB=Not Linked  CMPBUnits=Clock cycles  CMPBSource=Specify via dialog  CMPBValue_per=50  CMPBValue_clk=floor(target.PWM_Counter_Period/2+1)  enCMPBshadow=Counter equals to zero (CTR=Zero)  ePWMxLINKCMPC=Not Linked  CMPCUnits=Clock cycles  CMPCSource=Specify via dialog  CMPCValue_per=50  CMPCValue_clk=32000  enCMPCshadow=Counter equals to zero (CTR=Zero)  ePWMxLINKCMPD=Not Linked  CMPDUnits=Clock cycles  CMPDSource=Specify via dialog  CMPDValue_per=50  CMPDValue_clk=32000  enCMPDshadow=Counter equals to zero (CTR=Zero)  enableDBePWMxA=on  enableDBePWMxB=on  enhalfcycle=off  DBpolarity=Active high complementary (AHC)  DBedgeDelay=Positive  DBSource_ePWMxA=ePWMxA  DBSource_ePWMxB=ePWMxA  DBPeriodUnits=Clock cycles  DBperiodSource=Specify via dialog  REDperiod=15  FEDperiod=15  REDperiod_sec=0  FEDperiod_sec=0  LoadModeDBRED=Immediate without using shadow  LoadModeDBFED=Immediate without using shadow  adcstartModuleA=off  adcrequestEventA=First event  adcstartEventA=Digital Compare Module A Event 1 start of conversion (DCAEVT1.soc)  adcstartEventA_type2=Counter equals to period (CTR=PRD)  adcstartModuleB=off  adcrequestEventB=First event  adcstartEventB=Counter equals to zero (CTR=Zero)  adcstartEventB_type2=Counter equals to zero (CTR=Zero)  intEn=off  intPrd=First event  intSel=Counter equals to zero (CTR=Zero)  intSel_type2=Counter equals to zero (CTR=Zero)  hrpe=off  enHRPWM=off  HRPWM_LoadMode=Counter equals to period (CTR=PRD)  HRPWM_CTLMode=Duty or Period control mode  HRPWM_EDGMode=Both edge  hrpeb=off  enHRPWMB=off  HRPWM_LoadModeB=Counter equals to zero (CTR=ZERO)  HRPWM_CTLModeB=Duty or Period control mode  HRPWM_EDGModeB=Both edge  enHRDBRED=off  enHRDBFED=off  enSFO=on  enautoconv=on  chopperEnable=off  chopperFrequency=1  chopperFirstwidth=1  chopperDuty=12.5%  tripZonesource=Specify via dialog  tzselOSHT1=off  tzselOSHT2=off  tzselOSHT3=off  tzselOSHT4=off  tzselOSHT5=off  tzselOSHT6=off  tzselOSHDCAEV1=off  tzselOSHDCBEV1=off  tzselCBC1=off  tzselCBC2=off  tzselCBC3=off  tzselCBC4=off  tzselCBC5=off  tzselCBC6=off  tzselCBCDCAEV2=off  tzselCBCDCBEV2=off  enTzOstIntr=off  enTzCbcIntr=off  enTzDCAEVT1Intr=off  enTzDCAEVT2Intr=off  enTzDCBEVT1Intr=off  enTzDCBEVT2Intr=off  tzclrCBCLatch=Counter equals to zero (CTR=Zero)  ePWMxAforced=No action  ePWMxBforced=No action  DCAEVT1forced=No action  DCBEVT1forced=No action  DCAEVT2forced=No action  DCBEVT2forced=No action  dcah=Trip Zone 1 input (TZ1)  dcal=Trip Zone 2 input (TZ2)  dcbh=Trip Zone 1 input (TZ1)  dcbl=Trip Zone 2 input (TZ2)  dcah_type2=GPTRIP1SEL/(TZ1)  dcal_type2=GPTRIP2SEL/(TZ2)  dcbh_type2=GPTRIP1SEL/(TZ1)  dcbl_type2=GPTRIP2SEL/(TZ2)  gendcaevt1=Event disabled  gendcaevt2=Event disabled  gendcbevt1=Event disabled  gendcbevt2=Event disabled  dcaevt1src=DCAEVT1 with sync  dcaevt2src=DCAEVT2 with sync  dcbevt1src=DCBEVT1 with sync  dcbevt2src=DCBEVT2 with sync  pulsesel=Counter equals to zero (CTR=Zero)  blankinv=off  blankoffset=0  blankwidth=0  evsrcsel=Filtered version of DCAEVT1 (DCAEVT1FILT)  encape=off
  stop : Constant  Value=0  OutDataTypeStr=uint16
  DutyCycles : Outport  VectorParamsAs1DForOutWhenUnconnected=off
  wires:
  Demux1/3 -> ePWM3/1  "PWM_C"
  Scale_to_PWM_Counter_PRD/1 -> Switch1/1
  Mux2/1 -> Switch1/3
  stop/1 -> Mux2/3, Mux2/2, Mux2/1
  Inverter Signals/1 -> Demux/1
  Demux1/2 -> ePWM2/1  "PWM_B"
  Switch1/1 -> Demux1/1
  Demux1/1 -> ePWM1/1  "PWM_A"
  Mux/1 -> Scale_to_PWM_Counter_PRD/1  "PWM Duty Cycles"
  Ground/1 -> Mux1/1
  Ground1/1 -> Mux1/3
  Ground2/1 -> Mux1/2
  Mux1/1 -> DutyCycles/1
  Demux/1 -> Mux/1
  Demux/2 -> Mux/2
  Demux/3 -> Mux/3
  Constant/1 -> Switch/2
  NOT/1 -> Switch/3  "Active low logic for inverter enable"
  Demux/4 -> NOT/1, Switch/1, Switch1/2  "Active high logic for inverter enable"
  Switch/1 -> DRV830x Enable/1

== system mcb_pmsm_foc_sensorless_dyno_f28379d/FOC Algorithm Motor 1/Inverter (Simulation) ==
  Inverter Signals : Inport
  Data Type Duplicate : DataTypeDuplicate
  Demux : Demux
  Mux : Mux  Inputs=3
  Mux2 : Mux  Inputs=3
  Switch1 : Switch  Threshold=0.5  RndMeth=Simplest  SaturateOnIntegerOverflow=off  InputSameDT=off
  stop : Constant  Value=0  OutDataTypeStr=Inherit: Inherit via back propagation
  DutyCycles : Outport  VectorParamsAs1DForOutWhenUnconnected=off
  wires:
  stop/1 -> Data Type Duplicate/2, Mux2/1, Mux2/3, Mux2/2
  Mux2/1 -> Switch1/3
  Switch1/1 -> DutyCycles/1
  Inverter Signals/1 -> Demux/1
  Demux/4 -> Switch1/2  "PWM Enable"
  Mux/1 -> Data Type Duplicate/1, Switch1/1  "PWM Duty Cycles"
  Demux/1 -> Mux/1
  Demux/2 -> Mux/2
  Demux/3 -> Mux/3

== system mcb_pmsm_foc_sensorless_dyno_f28379d/FOC Algorithm Motor 1/Output Scaling ==
  Vabc_ref : Inport
  Constant : Constant  Value=0.5  OutDataTypeStr=dataType  SampleTime=-1
  Data Type Conversion : DataTypeConversion  OutDataTypeStr=dataType  SaturateOnIntegerOverflow=off  RndMeth=Floor
  Enable : DataStoreRead  DataStoreName=Enable  IndexOptions=Index vector (dialog)  Indices=1  OutputSizes=1
  One_by_Two : Gain  Gain=0.5  RndMeth=Simplest  OutDataTypeStr=Inherit: Same as input
  Sum : Sum  Inputs=|++
  PWM_Duty_Cycles : Outport
  PWM_Enable : Outport  Port=2
  wires:
  Constant/1 -> Sum/2
  Vabc_ref/1 -> One_by_Two/1
  Sum/1 -> PWM_Duty_Cycles/1  "PWM_Duty_Cycles"
  Enable/1 -> Data Type Conversion/1
  One_by_Two/1 -> Sum/1
  Data Type Conversion/1 -> PWM_Enable/1
